simulink model "rakka"  (R2021b)
settings: Solver=VariableStepAuto  StartTime=0.0  StopTime=10  RelTol=1e-3
values from neighbouring files (symbols this model uses):
  D = rho(2)    [tuning_ver2.m]
  I = rho(1)    [tuning_ver2.m]
  K = rho(3)    [tuning_ver2.m]
  omega_n = 10.3409    [tuning_ver2.m]
  t_Stance_Total = T_cycle * 0.62    (= 1.24)    [desire.m]
undefined symbols (not defined in the file or in its folder): K_d, theta
settings Model: Creator=KY  LastModifiedBy=KY

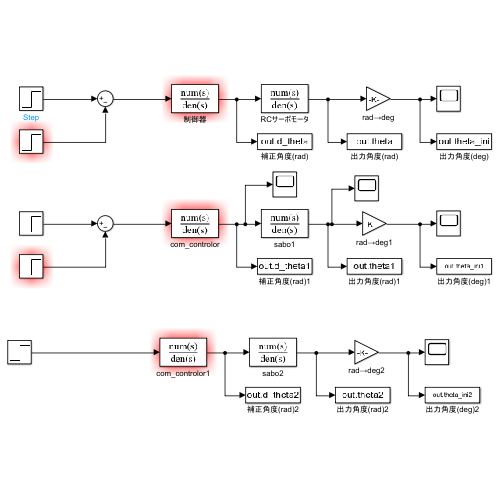
[thumbnail: Simulink's stored preview of the top-level diagram]
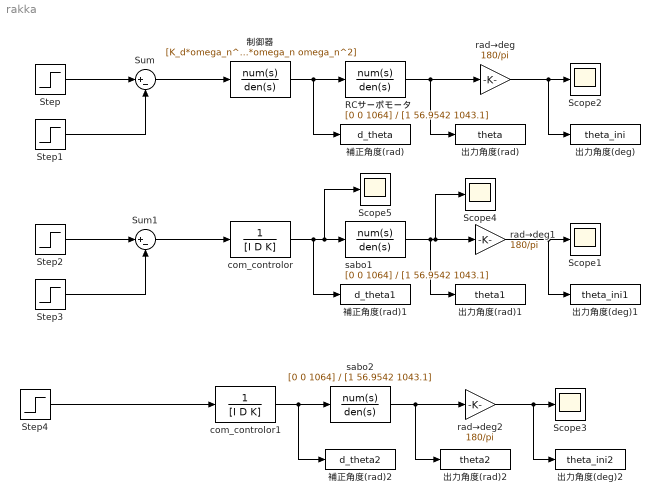
== system rakka ==
  RCサーボモータ : TransferFcn  Numerator=[0 0 1064]  Denominator=[1 56.9542 1043.1]
  Scope{1..5} (5 alike) : Scope
  Step : Step  After=0.43  SampleTime=0.001
  Step1 : Step  Time=1+t_Stance_Total  After=0.43  SampleTime=0.001
  Step2 : Step  After=0.43  SampleTime=0.001
  Step3 : Step  Time=1+t_Stance_Total  After=0.43  SampleTime=0.001
  Step4 : Step  After=0.43  SampleTime=0.001
  Sum : Sum  Inputs=|+-
  Sum1 : Sum  Inputs=|+-
  com_controlor : TransferFcn  Denominator=[I D K]
  com_controlor1 : TransferFcn  Denominator=[I D K]
  rad→deg : Gain  Gain=180/pi
  rad→deg1 : Gain  Gain=180/pi
  rad→deg2 : Gain  Gain=180/pi
  sabo1 : TransferFcn  Numerator=[0 0 1064]  Denominator=[1 56.9542 1043.1]
  sabo2 : TransferFcn  Numerator=[0 0 1064]  Denominator=[1 56.9542 1043.1]
  出力角度(deg) : ToWorkspace  VariableName=theta_ini  SaveFormat=Timeseries  SampleTime=-1
  出力角度(deg)1 : ToWorkspace  VariableName=theta_ini1  SaveFormat=Timeseries  SampleTime=-1
  出力角度(deg)2 : ToWorkspace  VariableName=theta_ini2  SaveFormat=Timeseries  SampleTime=-1
  出力角度(rad) : ToWorkspace  VariableName=theta  SaveFormat=Timeseries  SampleTime=-1
  出力角度(rad)1 : ToWorkspace  VariableName=theta1  SaveFormat=Timeseries  SampleTime=-1
  出力角度(rad)2 : ToWorkspace  VariableName=theta2  SaveFormat=Timeseries  SampleTime=-1
  制御器 : TransferFcn  Numerator=[K_d*omega_n^2]  Denominator=[1 2*theta*omega_n omega_n^2]
  補正角度(rad) : ToWorkspace  VariableName=d_theta  SaveFormat=Timeseries  SampleTime=0.001
  補正角度(rad)1 : ToWorkspace  VariableName=d_theta1  SaveFormat=Timeseries  SampleTime=0.001
  補正角度(rad)2 : ToWorkspace  VariableName=d_theta2  SaveFormat=Timeseries  SampleTime=0.001
  wires:
  rad→deg/1 -> 出力角度(deg)/1, Scope2/1
  制御器/1 -> RCサーボモータ/1, 補正角度(rad)/1
  RCサーボモータ/1 -> 出力角度(rad)/1, rad→deg/1
  Step1/1 -> Sum/2
  Step/1 -> Sum/1
  Sum/1 -> 制御器/1
  com_controlor/1 -> Scope5/1, sabo1/1, 補正角度(rad)1/1
  sabo1/1 -> 出力角度(rad)1/1, Scope4/1, rad→deg1/1
  rad→deg1/1 -> 出力角度(deg)1/1, Scope1/1
  Step2/1 -> Sum1/1
  Step3/1 -> Sum1/2
  Sum1/1 -> com_controlor/1
  Step4/1 -> com_controlor1/1
  rad→deg2/1 -> 出力角度(deg)2/1, Scope3/1
  com_controlor1/1 -> sabo2/1, 補正角度(rad)2/1
  sabo2/1 -> 出力角度(rad)2/1, rad→deg2/1
